simulink model "EleveinclinaisonLampe"  (R2018a)
settings: Solver=VariableStepAuto  StartTime=0.0  StopTime=0.3  RelTol=1e-3  EnableMultiTasking=on
undefined symbols (not defined in the file): articulation, biellette, biellette2, biellette_bati, biellette_reglage, derailleur_matlab, RootGround, RootPart
libraries: mblibv1 x20
settings Model: Creator=djellal  LastModifiedBy=Bennegen
settings DataIOCC: LimitDataPoints=on
settings OptimizationCC: LifeSpan=inf
settings DebuggingCC: AllowSymbolicDim=off  SFUnexpectedBacktrackingDiag=warning  SFNoUnconditionalDefaultTransitionDiag=warning  SFExecutionAtInitializationDiag=none
settings ModelReferenceCC: PropagateSignalLabelsOutOfModel=off
settings CodeAppCC: StateflowObjectComments=on
settings GRTTargetCC: TargetLangStandard=C89/C90 (ANSI)
settings ConfigComp: CovMetricSettings=dw  CovHtmlReporting=on  CovSaveCumulativeToWorkspaceVar=on  CovSaveSingleToWorkspaceVar=on  CovExternalEMLEnable=off
settings SimscapeCC: SimscapeNormalizeSystem=off
settings SimMechanicsCC: VisOnUpdateDiagram=on  VisDuringSimulation=on
settings ConfigurationSet: Description=SimMechanics 2G

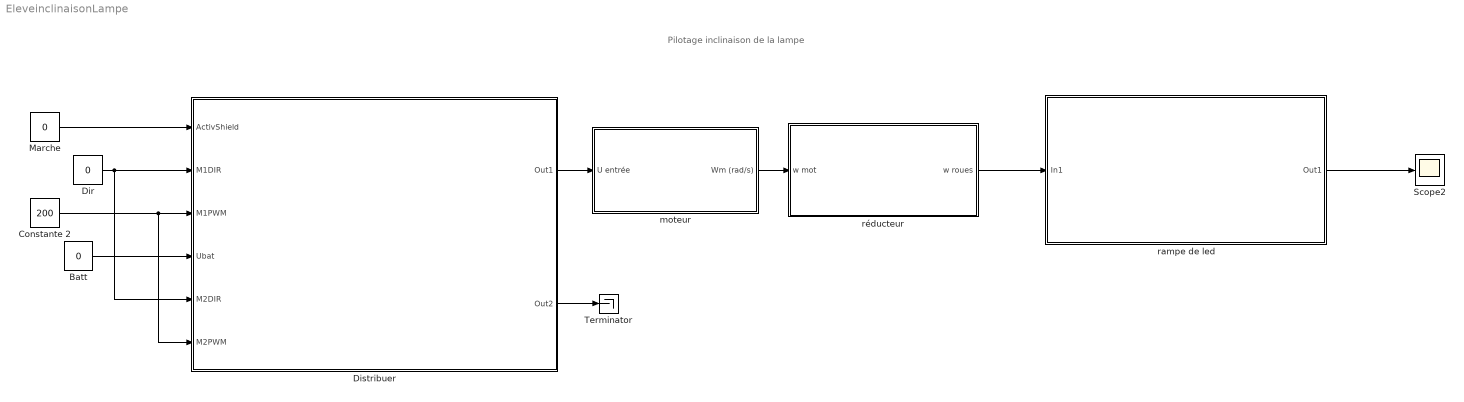
== system EleveinclinaisonLampe ==
  note: Pilotage inclinaison de la lampe
  Batt : Constant  Value=0  SampleTime=5
  Constante 2 : Constant  Value=200
  Dir : Constant  Value=0
  Distribuer : Subsystem
      mask Display:
      | image(imread('shieldMC33926.jpg'))
      | port_label('output', 1, 'Ushld1')
      | port_label('output', 2, 'Ushld2')
      | port_label('input', 1, 'Active')
      | port_label('input', 2, 'Dir1')
      | port_label('input', 3, 'PWM1')
      | port_label('input', 4, 'Ualim')
      | port_label('input', 5, 'Dir2')
      | port_label('input', 6, 'PWM2')
  "Marche " : Constant  Value=0
  Scope2 : Scope
  Terminator : Terminator
  moteur : Subsystem  mask{Ri=0, k=0, Cp=0, Jm=1e-5}
      mask prompts: Ri "R (Résistance induit en Ohm)"; k "k (Constante de vitesse(Vs/rad) ou de couple en N.m/A)"; Cp "Cp (Couple de pertes en N.m)"; Jm "Jm (Inertie moteur en kg.m²)"
      mask Display:
      | image(imread('moteur2.jpg'))
      | port_label('input', 1, 'U')
      | port_label('output', 1, 'wMot')
  rampe de led : Subsystem
      mask Display:
      | image('led.jpg')
      | port_label('input', 1, 'Vitesse angulaire')
      | port_label('output', 1, 'Position rampe LEDs')
  réducteur : Subsystem  mask{eta=0, k=0}
      mask prompts: eta "eta: rendement"; k "k: rapport de transmission"
      mask Display:
      | image(imread('reducteur2.jpg'))
      | port_label('input', 1, 'wMot')
      | port_label('output', 1, 'wRed')
  wires:
  Batt/1 -> Distribuer/4(Ubat)
  moteur/1(Wm (rad/s)) -> réducteur/1(w mot)
  "Marche "/1 -> Distribuer/1(ActivShield)
  Dir/1 -> Distribuer/2(M1DIR), Distribuer/5("M2DIR ")
  Distribuer/1(Out1) -> moteur/1(U entrée)
  Constante 2/1 -> Distribuer/6(M2PWM), Distribuer/3(M1PWM)
  Distribuer/2(Out2) -> Terminator/1
  réducteur/1(w roues) -> rampe de led/1(In1)
  rampe de led/1(Out1) -> Scope2/1

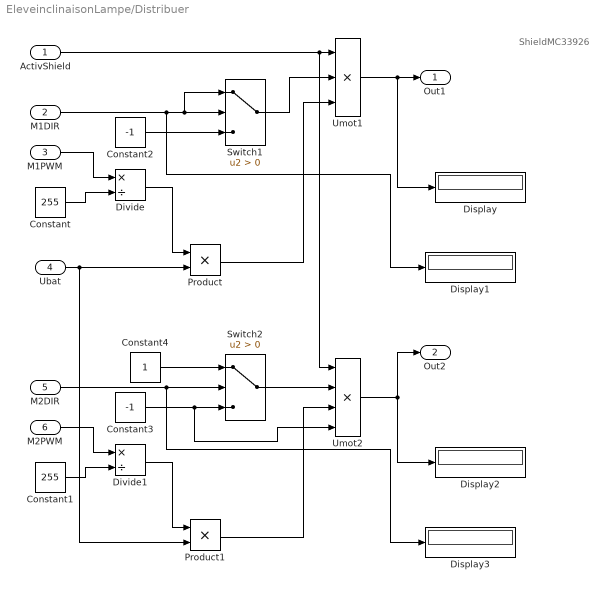
== system EleveinclinaisonLampe/Distribuer ==
  note: ShieldMC33926
  ActivShield : Inport
  M1DIR : Inport  Port=2
  M1PWM : Inport  Port=3
  Ubat : Inport  Port=4
  "M2DIR " : Inport  Port=5
  M2PWM : Inport  Port=6
  Constant : Constant  Value=255
  Constant1 : Constant  Value=255
  Constant2 : Constant  Value=-1
  Constant3 : Constant  Value=-1
  Constant4 : Constant
  Display{,1..3} (4 alike) : Display
  Divide : Product  Inputs=*/
  Divide1 : Product  Inputs=*/
  Product : Product
  Product1 : Product
  Switch1 : Switch  Criteria=u2 > Threshold
  Switch2 : Switch  Criteria=u2 > Threshold
  Umot1 : Product  Inputs=3
  Umot2 : Product  Inputs=4
  Out1 : Outport
  Out2 : Outport  Port=2
  wires:
  Ubat/1 -> Product1/2, Product/2
  M1PWM/1 -> Divide/1
  Constant/1 -> Divide/2
  Divide/1 -> Product/1
  Umot1/1 -> Display/1, Out1/1
  Product/1 -> Umot1/3
  M1DIR/1 -> Display1/1, Switch1/2, Switch1/1
  Constant2/1 -> Switch1/3
  Switch1/1 -> Umot1/2
  ActivShield/1 -> Umot2/1, Umot1/1
  M2PWM/1 -> Divide1/1
  Constant1/1 -> Divide1/2
  Divide1/1 -> Product1/1
  Umot2/1 -> Out2/1, Display2/1
  Product1/1 -> Umot2/3
  "M2DIR "/1 -> Display3/1, Switch2/2
  Constant3/1 -> Umot2/4, Switch2/3
  Switch2/1 -> Umot2/2
  Constant4/1 -> Switch2/1

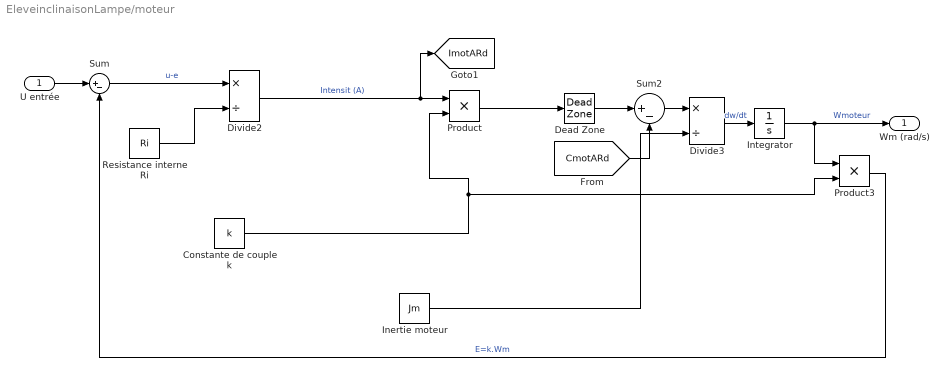
== system EleveinclinaisonLampe/moteur ==
  U entrée : Inport
  Constante de couple k : Constant  Value=k
  Dead Zone : DeadZone  LowerValue=-Cp  UpperValue=Cp  SaturateOnIntegerOverflow=on
  Divide2 : Product  Inputs=*/
  Divide3 : Product  Inputs=*/
  "Inertie moteur " : Constant  Value=Jm
  Integrator : Integrator
  Product : Product  RndMeth=Zero
  Product3 : Product  RndMeth=Zero
  Resistance interne Ri : Constant  Value=Ri
  Sum : Sum  Inputs=|+-
  Sum2 : Sum  Inputs=|+-
  Wm (rad/s) : Outport
  tag scope: ImotARd=global
  wires:
  Sum/1 -> Divide2/1  "u-e"
  Resistance interne Ri/1 -> Divide2/2
  Divide2/1 -> [ImotARd], Product/1  "Intensit (A)"
  Constante de couple k/1 -> Product/2, Product3/2
  "Inertie moteur "/1 -> Divide3/2
  Divide3/1 -> Integrator/1  "dw/dt"
  Integrator/1 -> Wm (rad/s)/1, Product3/1  "Wmoteur"
  Product3/1 -> Sum/2  "E=k.Wm"
  Dead Zone/1 -> Sum2/1
  Sum2/1 -> Divide3/1
  U entrée/1 -> Sum/1
  [CmotARd] -> Sum2/2
  Product/1 -> Dead Zone/1

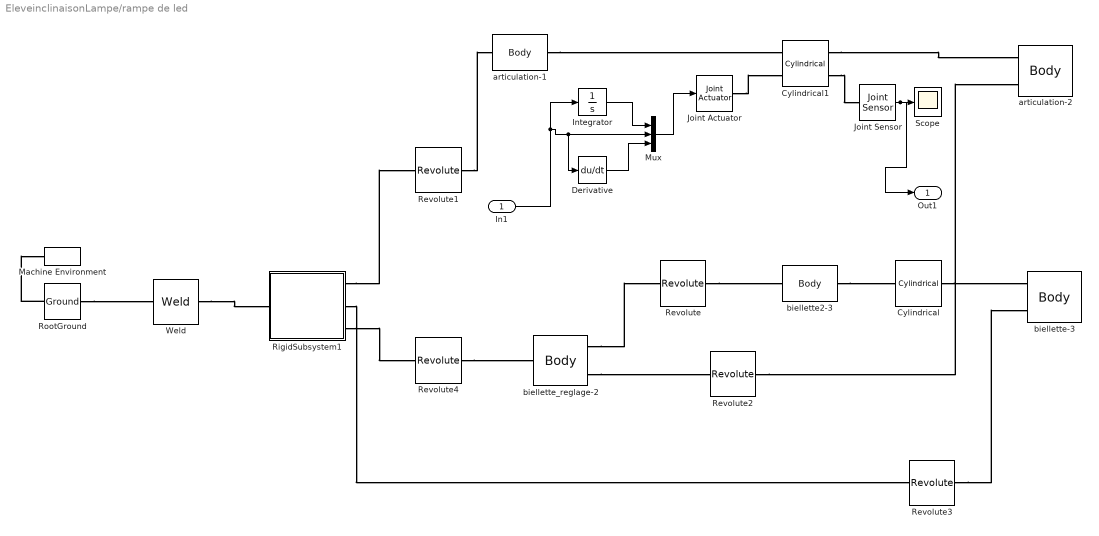
== system EleveinclinaisonLampe/rampe de led ==
  In1 : Inport
  Cylindrical : mblibv1/Joints/Cylindrical  LConnTagsString=__newl0  RConnTagsString=__newr0  UpdateFromCAD=on  PMImportedID=biellette-3:-:biellette2-3  NumSAPorts=0  CutJoint=off  MarkAsCut=off  Primitives=prismatic  PrimitiveProps=P1$WORLD$[0,0,-1]$prismatic#R1$WORLD$[0,0,1]$revolute  DialogClass=JointBlock  P1Axis=[0,0,-1]  R1Axis=[0,0,1]
      settings: SourceProductName=Simscape  SourceProductBaseCode=SS
  Cylindrical1 : mblibv1/Joints/Cylindrical  LConnTagsString=__newl0|SA1  RConnTagsString=__newr0|SA1  UpdateFromCAD=on  PMImportedID=articulation-1:-:articulation-2  NumSAPorts=2  CutJoint=off  MarkAsCut=off  Primitives=prismatic  PrimitiveProps=P1$World$[-0.575898,0.817522,0]$prismatic#R1$World$[-0.575898,0.817522,0]$revolute  DialogClass=JointBlock  P1Axis=[-0.575898,0.817522,0]  R1Axis=[-0.575898,0.817522,0]
      settings: SourceProductName=Simscape  SourceProductBaseCode=SS
  Derivative : Derivative
  Integrator : Integrator
  Joint Actuator : mblibv1/Sensors &  Actuators/Joint Actuator  UpdateFromCAD=off  PhysicalDomain=Mechanical  PortType=blob  ActuationStyle=Motion  AngleUnits=deg  ArcVelocityUnits=deg/s  ArcAccelerationUnits=deg/s^2  CoordPositionUnits=m  VelocityUnits=m/s  AccelerationUnits=m/s^2  ForceUnits=N  TorqueUnits=N*m  ActiveIO=on  Width=3  DialogClass=MechanicalActuatorBlock  Primitive=P1  ReferenceFrame=Absolute (World)
      settings: SourceProductName=Simscape  SourceProductBaseCode=SS
  Joint Sensor : mblibv1/Sensors &  Actuators/Joint Sensor  UpdateFromCAD=off  PhysicalDomain=Mechanical  PortType=blob  Muxed=on  Pose=off  Angle=on  AngleUnits=deg  ArcVelocity=off  ArcVelocityUnits=deg/s  ArcAcceleration=off  ArcAccelerationUnits=deg/s^2  CoordPosition=on  CoordPositionUnits=m  Velocity=off  VelocityUnits=m/s  Acceleration=off  AccelerationUnits=m/s^2  Quaternion=on  QuaternionDT=off  QuaternionDDT=off  QuaternionUnits=off  OutputVector=[1]  ActiveIO=on  Width=1  DialogClass=MechanicalSensorBlock  Primitive=P1  Force=off  ForceUnits=N  Torque=off  TorqueUnits=N-m  ReferenceFrame=Absolute (World)  ReactionSensedSide=Base  ReactionReferenceFrame=Absolute (World)  ReactionForce=off  ReactionForceUnits=N  ReactionMoment=off  ReactionMomentUnits=N-m
      settings: SourceProductName=Simscape  SourceProductBaseCode=SS
  Machine Environment : mblibv1/Bodies/Machine Environment  PortType=env  PhysicalDomain=Mechanical  DialogTemplateClass=MECH.MachineEnvironment  SyncWhenCopied=off  Gravity=[0 0 0]  GravityUnits=m/s^2  GravityAsSignal=off  Dimensionality=Auto-detect  AnalysisType=Forward dynamics  LinearAssemblyTolerance=1e-3  LinearAssemblyToleranceUnits=m  AngularAssemblyTolerance=1e-3  AngularAssemblyToleranceUnits=rad  ConstraintSolverType=Stabilizing  ConstraintRelTolerance=1e-4  ConstraintAbsTolerance=1e-4  UseRobustSingularityHandling=off  RedundancyAnalysisToleranceType=Automatically select tolerance  RedundancyAnalysisTolerance=1e-14  StatePerturbationType=Fixed  PerturbationSize=1e-5  VisualizeMachine=on  BodyVisualizationType=Use model default body geometries  BodyColorSelMode=Use model default  DefaultBodyColor=[1 0 0]
      settings: SourceProductName=Simscape  SourceProductBaseCode=SS
  Mux : Mux  Inputs=3
  Revolute : mblibv1/Joints/Revolute  LConnTagsString=__newl0  RConnTagsString=__newr0  UpdateFromCAD=on  PMImportedID=biellette2-3:-:biellette_reglage-2  NumSAPorts=0  CutJoint=off  MarkAsCut=off  Primitives=prismatic  PrimitiveProps=R1$WORLD$[0,0,-1]$revolute  DialogClass=JointBlock  R1Axis=[0,0,-1]
      settings: SourceProductName=Simscape  SourceProductBaseCode=SS
  Revolute1 : mblibv1/Joints/Revolute  LConnTagsString=__newl0  RConnTagsString=__newr0  UpdateFromCAD=on  PMImportedID=articulation-1:-:biellette_bati-1  NumSAPorts=0  CutJoint=off  MarkAsCut=off  Primitives=prismatic  PrimitiveProps=R1$WORLD$[0,0,1]$revolute  DialogClass=JointBlock  R1Axis=[0,0,1]
      settings: SourceProductName=Simscape  SourceProductBaseCode=SS
  Revolute2 : mblibv1/Joints/Revolute  LConnTagsString=__newl0  RConnTagsString=__newr0  UpdateFromCAD=on  PMImportedID=articulation-2:-:biellette_reglage-2  NumSAPorts=0  CutJoint=off  MarkAsCut=off  Primitives=prismatic  PrimitiveProps=R1$WORLD$[0,0,1]$revolute  DialogClass=JointBlock  R1Axis=[0,0,1]
      settings: SourceProductName=Simscape  SourceProductBaseCode=SS
  Revolute3 : mblibv1/Joints/Revolute  LConnTagsString=__newl0  RConnTagsString=__newr0  UpdateFromCAD=on  PMImportedID=biellette-3:-:biellette_bati-1  NumSAPorts=0  CutJoint=off  MarkAsCut=off  Primitives=prismatic  PrimitiveProps=R1$WORLD$[0,0,-1]$revolute  DialogClass=JointBlock  R1Axis=[0,0,-1]
      settings: SourceProductName=Simscape  SourceProductBaseCode=SS
  Revolute4 : mblibv1/Joints/Revolute  LConnTagsString=__newl0  RConnTagsString=__newr0  UpdateFromCAD=on  PMImportedID=biellette_bati-1:-:biellette_reglage-2  NumSAPorts=0  CutJoint=off  MarkAsCut=off  Primitives=prismatic  PrimitiveProps=R1$WORLD$[0,0,1]$revolute  DialogClass=JointBlock  R1Axis=[0,0,1]
      settings: SourceProductName=Simscape  SourceProductBaseCode=SS
  RigidSubsystem1 : Subsystem
      settings: MoveFcn=set_param(gcbh,'MaskDisplay','');set_param(gcbh,'MaskDisplay','mech_drawrigidss');
      mask Display: mech_drawrigidss
  RootGround : mblibv1/Bodies/Ground  UpdateFromCAD=on  PMImportedID=RootGround  LeftPortType=env  RightPortType=workingframe  PhysicalDomain=Mechanical  DialogClass=GroundBlock  CoordPosition=[0.00923858,-0.00722187,0.019358]  CoordPositionUnits=m  StateVectorMgrId=-1  MachineId=[0 0]  ShowEnvPort=on  ParameterChecksum=[4101816685, 1841262983, 2243035061, 1422340253]  TopologyChecksum=[3187384061, 3476322260, 1796620157, 391114162]
      settings: SourceProductName=Simscape  SourceProductBaseCode=SS
  Scope : Scope
  Weld : mblibv1/Joints/Weld  LConnTagsString=__newl0  RConnTagsString=__newr0  UpdateFromCAD=on  PMImportedID=RootGround:-:derailleur_matlab/RootPart  NumSAPorts=0  CutJoint=off  MarkAsCut=off  Primitives=weld  PrimitiveProps=W$WORLD$[0.57735,0.57735,0.57735]$weld  DialogClass=JointBlock  WAxis=[0.57735,0.57735,0.57735]
      settings: SourceProductName=Simscape  SourceProductBaseCode=SS
  articulation-1 : mblibv1/Bodies/Body  LConnTagsString=CS3  RConnTagsString=CS2  UpdateFromCAD=on  PMImportedID=articulation-1  DialogClass=MechanicalBodyBlock  Mass=5.85282e-05  MassUnits=kg  InertiaUnits=kg*m^2  Inertia=[2.77108e-10,1.37177e-15,4.41924e-17;1.37177e-15,2.894e-10,0;4.41924e-17,0,1.11426e-10]  Shape=Cylinder  ShapeDims=[1 1]  ShapeUnits=m  ShapeUse=false  Density=1  DensityUnits=kg/m^3  DensityUse=false  GraphicsMode=GFXFILE  GraphicsFileName=derailleur_matlab - articulation-1.STL  BodyColorSelMode=COLORPALETTE  BodyColor=[1;0.501961;1]  AttachedToCS=CS1  CG=Right$CG$[-0.00835506 0.0121026 0.025871]$WORLD$WORLD$m$[0.817522 -0.575898 0;0.575898 0.817522 0;0 0 1]$3x3 Transform$rad$WORLD$false$articulation-1::CG(AUTOGEN)  WorkingFrames=Right$CS1$[-0.00835506 0.0121026 0.0213743]$WORLD$WORLD$m$[0.817522 -0.575898 0;0.575898 0.817522 0;0 0 1]$3x3 Transform$rad$WORLD$false$articulation-1::CS1(AUTOGEN)#Right$CS2$[0.00460264 -0.0062916 0.0263743]$WORLD$WORLD$m$[1 0 0;0 1 0;0 0 1]$3x3 Transform$rad$WORLD$true$articulation-1:-:articulation-2::articulation-1(AUTOGEN)#Left$CS3$[-0.00835506 0.0121026 0.0238743]$WORLD$WORLD$m$[1 0 0;0 1 0;0 0 1]$3x3 Transform$rad$WORLD$true$articulation-1:-:biellette_bati-1::articulation-1(AUTOGEN)  CGPos=[-0.00835506 0.0121026 0.025871]  CGRot=[0.817522 -0.575898 0;0.575898 0.817522 0;0 0 1]  CS0Pos=[]  CS0Rot=[]  CS1Pos=[-0.00835506 0.0121026 0.0213743]  CS1Rot=[0.817522 -0.575898 0;0.575898 0.817522 0;0 0 1]  CS2Pos=[0.00460264 -0.0062916 0.0263743]  CS2Rot=[1 0 0;0 1 0;0 0 1]  CS3Pos=[-0.00835506 0.0121026 0.0238743]  CS3Rot=[1 0 0;0 1 0;0 0 1]  CS4Pos=[]  CS4Rot=[]  CS5Pos=[]  CS5Rot=[]  CS6Pos=[]  CS6Rot=[]  CS7Pos=[]  CS7Rot=[]  CS8Pos=[]  CS8Rot=[]  CS9Pos=[]  CS9Rot=[]  CS10Pos=[]  CS10Rot=[]  CS11Pos=[]  CS11Rot=[]  CS12Pos=[]  CS12Rot=[]  CS13Pos=[]  CS13Rot=[]  CS14Pos=[]  CS14Rot=[]  CS15Pos=[]  CS15Rot=[]  CS16Pos=[]  CS16Rot=[]  CS17Pos=[]  CS17Rot=[]  CS18Pos=[]  CS18Rot=[]  CS19Pos=[]  CS19Rot=[]  CS20Pos=[]  CS20Rot=[]
      settings: SourceProductName=Simscape  SourceProductBaseCode=SS
  articulation-2 : mblibv1/Bodies/Body  LConnTagsString=CS2|CS3  UpdateFromCAD=on  PMImportedID=articulation-2  DialogClass=MechanicalBodyBlock  Mass=5.85282e-05  MassUnits=kg  InertiaUnits=kg*m^2  Inertia=[2.77108e-10,1.37177e-15,4.41924e-17;1.37177e-15,2.894e-10,0;4.41924e-17,0,1.11426e-10]  Shape=Cylinder  ShapeDims=[1 1]  ShapeUnits=m  ShapeUse=false  Density=1  DensityUnits=kg/m^3  DensityUse=false  GraphicsMode=GFXFILE  GraphicsFileName=derailleur_matlab - articulation-2.STL  BodyColorSelMode=COLORPALETTE  BodyColor=[1;0.501961;1]  AttachedToCS=CS1  CG=Right$CG$[0.00945682 -0.0131824 0.025871]$WORLD$WORLD$m$[0.817522 -0.575898 0;0.575898 0.817522 0;0 0 1]$3x3 Transform$rad$WORLD$false$articulation-2::CG(AUTOGEN)  WorkingFrames=Right$CS1$[0.00945682 -0.0131824 0.0213743]$WORLD$WORLD$m$[0.817522 -0.575898 0;0.575898 0.817522 0;0 0 1]$3x3 Transform$rad$WORLD$false$articulation-2::CS1(AUTOGEN)#Left$CS2$[0.00460264 -0.0062916 0.0263743]$WORLD$WORLD$m$[1 0 0;0 1 0;0 0 1]$3x3 Transform$rad$WORLD$true$articulation-1:-:articulation-2::articulation-2(AUTOGEN)#Left$CS3$[0.00945682 -0.0131824 0.0163743]$WORLD$WORLD$m$[1 0 0;0 1 0;0 0 1]$3x3 Transform$rad$WORLD$true$articulation-2:-:biellette_reglage-2::articulation-2(AUTOGEN)  CGPos=[0.00945682 -0.0131824 0.025871]  CGRot=[0.817522 -0.575898 0;0.575898 0.817522 0;0 0 1]  CS0Pos=[]  CS0Rot=[]  CS1Pos=[0.00945682 -0.0131824 0.0213743]  CS1Rot=[0.817522 -0.575898 0;0.575898 0.817522 0;0 0 1]  CS2Pos=[0.00460264 -0.0062916 0.0263743]  CS2Rot=[1 0 0;0 1 0;0 0 1]  CS3Pos=[0.00945682 -0.0131824 0.0163743]  CS3Rot=[1 0 0;0 1 0;0 0 1]  CS4Pos=[]  CS4Rot=[]  CS5Pos=[]  CS5Rot=[]  CS6Pos=[]  CS6Rot=[]  CS7Pos=[]  CS7Rot=[]  CS8Pos=[]  CS8Rot=[]  CS9Pos=[]  CS9Rot=[]  CS10Pos=[]  CS10Rot=[]  CS11Pos=[]  CS11Rot=[]  CS12Pos=[]  CS12Rot=[]  CS13Pos=[]  CS13Rot=[]  CS14Pos=[]  CS14Rot=[]  CS15Pos=[]  CS15Rot=[]  CS16Pos=[]  CS16Rot=[]  CS17Pos=[]  CS17Rot=[]  CS18Pos=[]  CS18Rot=[]  CS19Pos=[]  CS19Rot=[]  CS20Pos=[]  CS20Rot=[]
      settings: SourceProductName=Simscape  SourceProductBaseCode=SS
  biellette-3 : mblibv1/Bodies/Body  LConnTagsString=CS2|CS3  UpdateFromCAD=on  PMImportedID=biellette-3  DialogClass=MechanicalBodyBlock  Mass=0.00106676  MassUnits=kg  InertiaUnits=kg*m^2  Inertia=[1.66571e-07,0,0;0,4.45129e-09,0;0,0,1.66578e-07]  Shape=Cylinder  ShapeDims=[1 1]  ShapeUnits=m  ShapeUse=false  Density=1  DensityUnits=kg/m^3  DensityUse=false  GraphicsMode=GFXFILE  GraphicsFileName=derailleur_matlab - biellette-3.STL  BodyColorSelMode=COLORPALETTE  BodyColor=[0;1;1]  AttachedToCS=CS1  CG=Right$CG$[0.0011179 -0.00759352 0.0188743]$WORLD$WORLD$m$[0.984808 -0.173648 0;0.173648 0.984808 0;0 0 1]$3x3 Transform$rad$WORLD$false$biellette-3::CG(AUTOGEN)  WorkingFrames=Right$CS1$[0.00459087 -0.0272897 0.0163743]$WORLD$WORLD$m$[0.984808 -0.173648 0;0.173648 0.984808 0;0 0 1]$3x3 Transform$rad$WORLD$false$biellette-3::CS1(AUTOGEN)#Left$CS2$[0.00459087 -0.0272897 0.0138743]$WORLD$WORLD$m$[1 0 0;0 1 0;0 0 1]$3x3 Transform$rad$WORLD$true$biellette-3:-:biellette2-3::biellette-3(AUTOGEN)#Left$CS3$[-0.00235506 0.0121026 0.0238743]$WORLD$WORLD$m$[1 0 0;0 1 0;0 0 1]$3x3 Transform$rad$WORLD$true$biellette-3:-:biellette_bati-1::biellette-3(AUTOGEN)  CGPos=[0.0011179 -0.00759352 0.0188743]  CGRot=[0.984808 -0.173648 0;0.173648 0.984808 0;0 0 1]  CS0Pos=[]  CS0Rot=[]  CS1Pos=[0.00459087 -0.0272897 0.0163743]  CS1Rot=[0.984808 -0.173648 0;0.173648 0.984808 0;0 0 1]  CS2Pos=[0.00459087 -0.0272897 0.0138743]  CS2Rot=[1 0 0;0 1 0;0 0 1]  CS3Pos=[-0.00235506 0.0121026 0.0238743]  CS3Rot=[1 0 0;0 1 0;0 0 1]  CS4Pos=[]  CS4Rot=[]  CS5Pos=[]  CS5Rot=[]  CS6Pos=[]  CS6Rot=[]  CS7Pos=[]  CS7Rot=[]  CS8Pos=[]  CS8Rot=[]  CS9Pos=[]  CS9Rot=[]  CS10Pos=[]  CS10Rot=[]  CS11Pos=[]  CS11Rot=[]  CS12Pos=[]  CS12Rot=[]  CS13Pos=[]  CS13Rot=[]  CS14Pos=[]  CS14Rot=[]  CS15Pos=[]  CS15Rot=[]  CS16Pos=[]  CS16Rot=[]  CS17Pos=[]  CS17Rot=[]  CS18Pos=[]  CS18Rot=[]  CS19Pos=[]  CS19Rot=[]  CS20Pos=[]  CS20Rot=[]
      settings: SourceProductName=Simscape  SourceProductBaseCode=SS
  biellette2-3 : mblibv1/Bodies/Body  LConnTagsString=CS3  RConnTagsString=CS2  UpdateFromCAD=on  PMImportedID=biellette2-3  DialogClass=MechanicalBodyBlock  Mass=0.000699161  MassUnits=kg  InertiaUnits=kg*m^2  Inertia=[1.15213e-08,0,0;0,3.54087e-08,0;0,0,2.85179e-08]  Shape=Cylinder  ShapeDims=[1 1]  ShapeUnits=m  ShapeUse=false  Density=1  DensityUnits=kg/m^3  DensityUse=false  GraphicsMode=GFXFILE  GraphicsFileName=derailleur_matlab - biellette2-3.STL  BodyColorSelMode=COLORPALETTE  BodyColor=[0;1;0]  AttachedToCS=CS1  CG=Right$CG$[0.0130909 -0.027583 0.0188743]$WORLD$WORLD$m$[1 0 0;0 -1 0;0 0 -1]$3x3 Transform$rad$WORLD$false$biellette2-3::CG(AUTOGEN)  WorkingFrames=Right$CS1$[0.00459087 -0.0272897 0.0188743]$WORLD$WORLD$m$[1 0 0;0 -1 0;0 0 -1]$3x3 Transform$rad$WORLD$false$biellette2-3::CS1(AUTOGEN)#Right$CS2$[0.00459087 -0.0272897 0.0138743]$WORLD$WORLD$m$[1 0 0;0 1 0;0 0 1]$3x3 Transform$rad$WORLD$true$biellette-3:-:biellette2-3::biellette2-3(AUTOGEN)#Left$CS3$[0.0215909 -0.0272897 0.0213743]$WORLD$WORLD$m$[1 0 0;0 1 0;0 0 1]$3x3 Transform$rad$WORLD$true$biellette2-3:-:biellette_reglage-2::biellette2-3(AUTOGEN)  CGPos=[0.0130909 -0.027583 0.0188743]  CGRot=[1 0 0;0 -1 0;0 0 -1]  CS0Pos=[]  CS0Rot=[]  CS1Pos=[0.00459087 -0.0272897 0.0188743]  CS1Rot=[1 0 0;0 -1 0;0 0 -1]  CS2Pos=[0.00459087 -0.0272897 0.0138743]  CS2Rot=[1 0 0;0 1 0;0 0 1]  CS3Pos=[0.0215909 -0.0272897 0.0213743]  CS3Rot=[1 0 0;0 1 0;0 0 1]  CS4Pos=[]  CS4Rot=[]  CS5Pos=[]  CS5Rot=[]  CS6Pos=[]  CS6Rot=[]  CS7Pos=[]  CS7Rot=[]  CS8Pos=[]  CS8Rot=[]  CS9Pos=[]  CS9Rot=[]  CS10Pos=[]  CS10Rot=[]  CS11Pos=[]  CS11Rot=[]  CS12Pos=[]  CS12Rot=[]  CS13Pos=[]  CS13Rot=[]  CS14Pos=[]  CS14Rot=[]  CS15Pos=[]  CS15Rot=[]  CS16Pos=[]  CS16Rot=[]  CS17Pos=[]  CS17Rot=[]  CS18Pos=[]  CS18Rot=[]  CS19Pos=[]  CS19Rot=[]  CS20Pos=[]  CS20Rot=[]
      settings: SourceProductName=Simscape  SourceProductBaseCode=SS
  biellette_reglage-2 : mblibv1/Bodies/Body  LConnTagsString=CS4  RConnTagsString=CS2|CS3  UpdateFromCAD=on  PMImportedID=biellette_reglage-2  DialogClass=MechanicalBodyBlock  Mass=0.00127425  MassUnits=kg  InertiaUnits=kg*m^2  Inertia=[1.72519e-07,-3.13484e-09,2.93891e-09;-3.13484e-09,1.40927e-08,2.60554e-09;2.93891e-09,2.60554e-09,1.77065e-07]  Shape=Cylinder  ShapeDims=[1 1]  ShapeUnits=m  ShapeUse=false  Density=1  DensityUnits=kg/m^3  DensityUse=false  GraphicsMode=GFXFILE  GraphicsFileName=derailleur_matlab - biellette_reglage-2.STL  BodyColorSelMode=COLORPALETTE  BodyColor=[1;0;0]  AttachedToCS=CS1  CG=Right$CG$[0.0175075 -0.00836253 0.0194849]$WORLD$WORLD$m$[0.984808 -0.173648 0;0.173648 0.984808 0;0 0 1]$3x3 Transform$rad$WORLD$false$biellette_reglage-2::CG(AUTOGEN)  WorkingFrames=Right$CS1$[0.0215909 -0.0272897 0.0163743]$WORLD$WORLD$m$[0.984808 -0.173648 0;0.173648 0.984808 0;0 0 1]$3x3 Transform$rad$WORLD$false$biellette_reglage-2::CS1(AUTOGEN)#Right$CS2$[0.0215909 -0.0272897 0.0213743]$WORLD$WORLD$m$[1 0 0;0 1 0;0 0 1]$3x3 Transform$rad$WORLD$true$biellette2-3:-:biellette_reglage-2::biellette_reglage-2(AUTOGEN)#Right$CS3$[0.00945682 -0.0131824 0.0163743]$WORLD$WORLD$m$[1 0 0;0 1 0;0 0 1]$3x3 Transform$rad$WORLD$true$articulation-2:-:biellette_reglage-2::biellette_reglage-2(AUTOGEN)#Left$CS4$[0.0146449 0.0121026 0.0163743]$WORLD$WORLD$m$[1 0 0;0 1 0;0 0 1]$3x3 Transform$rad$WORLD$true$biellette_bati-1:-:biellette_reglage-2::biellette_reglage-2(AUTOGEN)  CGPos=[0.0175075 -0.00836253 0.0194849]  CGRot=[0.984808 -0.173648 0;0.173648 0.984808 0;0 0 1]  CS0Pos=[]  CS0Rot=[]  CS1Pos=[0.0215909 -0.0272897 0.0163743]  CS1Rot=[0.984808 -0.173648 0;0.173648 0.984808 0;0 0 1]  CS2Pos=[0.0215909 -0.0272897 0.0213743]  CS2Rot=[1 0 0;0 1 0;0 0 1]  CS3Pos=[0.00945682 -0.0131824 0.0163743]  CS3Rot=[1 0 0;0 1 0;0 0 1]  CS4Pos=[0.0146449 0.0121026 0.0163743]  CS4Rot=[1 0 0;0 1 0;0 0 1]  CS5Pos=[]  CS5Rot=[]  CS6Pos=[]  CS6Rot=[]  CS7Pos=[]  CS7Rot=[]  CS8Pos=[]  CS8Rot=[]  CS9Pos=[]  CS9Rot=[]  CS10Pos=[]  CS10Rot=[]  CS11Pos=[]  CS11Rot=[]  CS12Pos=[]  CS12Rot=[]  CS13Pos=[]  CS13Rot=[]  CS14Pos=[]  CS14Rot=[]  CS15Pos=[]  CS15Rot=[]  CS16Pos=[]  CS16Rot=[]  CS17Pos=[]  CS17Rot=[]  CS18Pos=[]  CS18Rot=[]  CS19Pos=[]  CS19Rot=[]  CS20Pos=[]  CS20Rot=[]
      settings: SourceProductName=Simscape  SourceProductBaseCode=SS
  Out1 : Outport
  wires:
  Joint Sensor/1 -> Out1/1, Scope/1
  Derivative/1 -> Mux/3
  In1/1 -> Integrator/1, Derivative/1, Mux/2
  Integrator/1 -> Mux/1
  Mux/1 -> Joint Actuator/1
  connections:
  Cylindrical1/RConn1 -- articulation-2/LConn1
  articulation-1/RConn1 -- Cylindrical1/LConn1
  Cylindrical1/RConn2 -- Joint Sensor/LConn1
  Joint Actuator/RConn1 -- Cylindrical1/LConn2
  RootGround/LConn1 -- Machine Environment/RConn1
  Weld/RConn1 -- RigidSubsystem1/LConn1
  Revolute4/RConn1 -- biellette_reglage-2/LConn1
  RigidSubsystem1/RConn3 -- Revolute4/LConn1
  Revolute3/RConn1 -- biellette-3/LConn2
  RigidSubsystem1/RConn2 -- Revolute3/LConn1
  biellette_reglage-2/RConn2 -- Revolute2/LConn1
  Revolute1/RConn1 -- articulation-1/LConn1
  Revolute2/RConn1 -- articulation-2/LConn2
  RigidSubsystem1/RConn1 -- Revolute1/LConn1
  Cylindrical/RConn1 -- biellette-3/LConn1
  Revolute/RConn1 -- biellette2-3/LConn1
  biellette_reglage-2/RConn1 -- Revolute/LConn1
  biellette2-3/RConn1 -- Cylindrical/LConn1
  RootGround/RConn1 -- Weld/LConn1

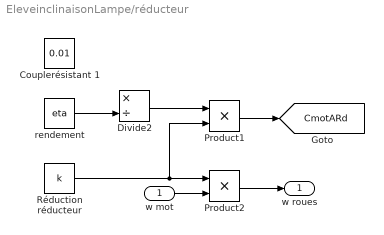
== system EleveinclinaisonLampe/réducteur ==
  w mot : Inport
  Couplerésistant 1 : Constant  Value=0.01  VectorParams1D=off
  Divide2 : Product  Inputs=*/
  Product1 : Product  RndMeth=Zero
  Product2 : Product  Inputs=**
  Réduction réducteur : Constant  Value=k
  "rendement " : Constant  Value=eta  VectorParams1D=off
  w roues : Outport
  tag scope: CmotARd=global
  wires:
  Réduction réducteur/1 -> Product2/1, Product1/2
  w mot/1 -> Product2/2
  Product2/1 -> w roues/1
  "rendement "/1 -> Divide2/2
  Divide2/1 -> Product1/1
  ? -> Divide2/1
  Product1/1 -> [CmotARd]

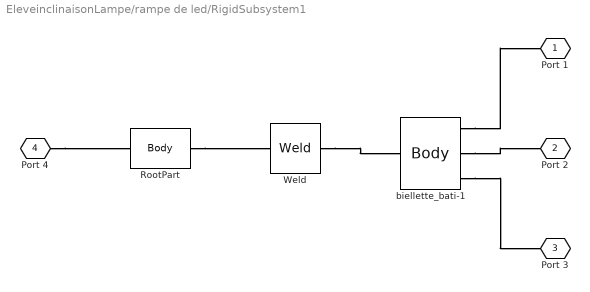
== system EleveinclinaisonLampe/rampe de led/RigidSubsystem1 ==
  RootPart : mblibv1/Bodies/Body  LConnTagsString=CS3  RConnTagsString=CS2  UpdateFromCAD=on  PMImportedID=derailleur_matlab/RootPart  DialogClass=MechanicalBodyBlock  Mass=0  MassUnits=kg  InertiaUnits=kg*m^2  Inertia=[0,0,0;0,0,0;0,0,0]  Shape=Cylinder  ShapeDims=[1 1]  ShapeUnits=m  ShapeUse=false  Density=1  DensityUnits=kg/m^3  DensityUse=false  GraphicsMode=MACHINE_DEFAULT  BodyColorSelMode=MACHINE_DEFAULT  BodyColor=[1;0;0]  AttachedToCS=CS1  CG=Right$CG$[0.00923858 -0.00722187 0.019358]$WORLD$WORLD$m$[1 0 0;0 1 0;0 0 1]$3x3 Transform$rad$WORLD$false$derailleur_matlab/RootPart::CG(AUTOGEN)  WorkingFrames=Right$CS1$[0 0 0]$WORLD$WORLD$m$[1 0 0;0 1 0;0 0 1]$3x3 Transform$rad$WORLD$false$derailleur_matlab/RootPart::CS1(AUTOGEN)#Right$CS2$[0.00469458 0.0123651 0.0192686]$WORLD$WORLD$m$[1 0 0;0 1 0;0 0 1]$3x3 Transform$rad$WORLD$true$biellette_bati-1:-:derailleur_matlab/RootPart::derailleur_matlab/RootPart(AUTOGEN)#Left$CS3$[0.00923858 -0.00722187 0.019358]$WORLD$WORLD$m$[1 0 0;0 1 0;0 0 1]$3x3 Transform$rad$WORLD$true$RootGround:-:derailleur_matlab/RootPart::derailleur_matlab/RootPart(AUTOGEN)  CGPos=[0.00923858 -0.00722187 0.019358]  CGRot=[1 0 0;0 1 0;0 0 1]  CS0Pos=[]  CS0Rot=[]  CS1Pos=[0 0 0]  CS1Rot=[1 0 0;0 1 0;0 0 1]  CS2Pos=[0.00469458 0.0123651 0.0192686]  CS2Rot=[1 0 0;0 1 0;0 0 1]  CS3Pos=[0.00923858 -0.00722187 0.019358]  CS3Rot=[1 0 0;0 1 0;0 0 1]  CS4Pos=[]  CS4Rot=[]  CS5Pos=[]  CS5Rot=[]  CS6Pos=[]  CS6Rot=[]  CS7Pos=[]  CS7Rot=[]  CS8Pos=[]  CS8Rot=[]  CS9Pos=[]  CS9Rot=[]  CS10Pos=[]  CS10Rot=[]  CS11Pos=[]  CS11Rot=[]  CS12Pos=[]  CS12Rot=[]  CS13Pos=[]  CS13Rot=[]  CS14Pos=[]  CS14Rot=[]  CS15Pos=[]  CS15Rot=[]  CS16Pos=[]  CS16Rot=[]  CS17Pos=[]  CS17Rot=[]  CS18Pos=[]  CS18Rot=[]  CS19Pos=[]  CS19Rot=[]  CS20Pos=[]  CS20Rot=[]
      settings: SourceProductName=Simscape  SourceProductBaseCode=SS
  Weld : mblibv1/Joints/Weld  LConnTagsString=__newl0  RConnTagsString=__newr0  UpdateFromCAD=on  PMImportedID=biellette_bati-1:-:derailleur_matlab/RootPart  NumSAPorts=0  CutJoint=off  MarkAsCut=off  Primitives=weld  PrimitiveProps=W$WORLD$[0.57735,0.57735,0.57735]$weld  DialogClass=JointBlock  WAxis=[0.57735,0.57735,0.57735]
      settings: SourceProductName=Simscape  SourceProductBaseCode=SS
  biellette_bati-1 : mblibv1/Bodies/Body  LConnTagsString=CS2  RConnTagsString=CS3|CS4|CS5  UpdateFromCAD=on  PMImportedID=biellette_bati-1  DialogClass=MechanicalBodyBlock  Mass=0.000781307  MassUnits=kg  InertiaUnits=kg*m^2  Inertia=[1.28722e-08,-2.97443e-10,3.80263e-09;-2.97443e-10,5.07782e-08,8.08583e-11;3.80263e-09,8.08583e-11,4.30853e-08]  Shape=Cylinder  ShapeDims=[1 1]  ShapeUnits=m  ShapeUse=false  Density=1  DensityUnits=kg/m^3  DensityUse=false  GraphicsMode=GFXFILE  GraphicsFileName=derailleur_matlab - biellette_bati-1.STL  BodyColorSelMode=COLORPALETTE  BodyColor=[0.792157;0.819608;0.933333]  AttachedToCS=CS1  CG=Right$CG$[0.00469458 0.0123651 0.0192686]$WORLD$WORLD$m$[1 0 0;0 1 0;0 0 1]$3x3 Transform$rad$WORLD$false$biellette_bati-1::CG(AUTOGEN)  WorkingFrames=Right$CS1$[-0.00235506 0.0121026 0.0188743]$WORLD$WORLD$m$[1 0 0;0 1 0;0 0 1]$3x3 Transform$rad$WORLD$false$biellette_bati-1::CS1(AUTOGEN)#Left$CS2$[0.00469458 0.0123651 0.0192686]$WORLD$WORLD$m$[1 0 0;0 1 0;0 0 1]$3x3 Transform$rad$WORLD$true$biellette_bati-1:-:derailleur_matlab/RootPart::biellette_bati-1(AUTOGEN)#Right$CS3$[-0.00835506 0.0121026 0.0238743]$WORLD$WORLD$m$[1 0 0;0 1 0;0 0 1]$3x3 Transform$rad$WORLD$true$articulation-1:-:biellette_bati-1::biellette_bati-1(AUTOGEN)#Right$CS4$[-0.00235506 0.0121026 0.0238743]$WORLD$WORLD$m$[1 0 0;0 1 0;0 0 1]$3x3 Transform$rad$WORLD$true$biellette-3:-:biellette_bati-1::biellette_bati-1(AUTOGEN)#Right$CS5$[0.0146449 0.0121026 0.0163743]$WORLD$WORLD$m$[1 0 0;0 1 0;0 0 1]$3x3 Transform$rad$WORLD$true$biellette_bati-1:-:biellette_reglage-2::biellette_bati-1(AUTOGEN)  CGPos=[0.00469458 0.0123651 0.0192686]  CGRot=[1 0 0;0 1 0;0 0 1]  CS0Pos=[]  CS0Rot=[]  CS1Pos=[-0.00235506 0.0121026 0.0188743]  CS1Rot=[1 0 0;0 1 0;0 0 1]  CS2Pos=[0.00469458 0.0123651 0.0192686]  CS2Rot=[1 0 0;0 1 0;0 0 1]  CS3Pos=[-0.00835506 0.0121026 0.0238743]  CS3Rot=[1 0 0;0 1 0;0 0 1]  CS4Pos=[-0.00235506 0.0121026 0.0238743]  CS4Rot=[1 0 0;0 1 0;0 0 1]  CS5Pos=[0.0146449 0.0121026 0.0163743]  CS5Rot=[1 0 0;0 1 0;0 0 1]  CS6Pos=[]  CS6Rot=[]  CS7Pos=[]  CS7Rot=[]  CS8Pos=[]  CS8Rot=[]  CS9Pos=[]  CS9Rot=[]  CS10Pos=[]  CS10Rot=[]  CS11Pos=[]  CS11Rot=[]  CS12Pos=[]  CS12Rot=[]  CS13Pos=[]  CS13Rot=[]  CS14Pos=[]  CS14Rot=[]  CS15Pos=[]  CS15Rot=[]  CS16Pos=[]  CS16Rot=[]  CS17Pos=[]  CS17Rot=[]  CS18Pos=[]  CS18Rot=[]  CS19Pos=[]  CS19Rot=[]  CS20Pos=[]  CS20Rot=[]
      settings: SourceProductName=Simscape  SourceProductBaseCode=SS
  Port 1 : PMIOPort  Side=Right
  Port 2 : PMIOPort  Port=2  Side=Right
  Port 3 : PMIOPort  Port=3  Side=Right
  Port 4 : PMIOPort  Port=4  Side=Left
  connections:
  RootPart/RConn1 -- Weld/LConn1
  Weld/RConn1 -- biellette_bati-1/LConn1
  biellette_bati-1/RConn1 -- Port 1/RConn1
  biellette_bati-1/RConn2 -- Port 2/RConn1
  biellette_bati-1/RConn3 -- Port 3/RConn1
  Port 4/RConn1 -- RootPart/LConn1
